simulink model "Alternative_VTOLAutopilotController"  (R2026a)
settings: configuration reference "VTOLConfiguration" (kept outside this file)
undefined symbols (not defined in the file): control, controlParams, ControlSampleTime, CriticalTiltAngle, DiscIntNeverNeededParam, dspblkCoreblockFVToolHelper, flightState, FSState, FWControlParams, FWTrimSpeed, gcbh, R_LOOKAHEAD, ReferenceFilterDen, ReferenceFilterNum, tilt_max, tilt_trim, tiltIni, TiltScheduleRate, uavParam, Vt, w_trim, WindDownRate, zGround
libraries: slpidlib x31, simulink x10, uavalgslib x7, simulink_extras x1, sl_discontinuities x1
(part 3 of 6)

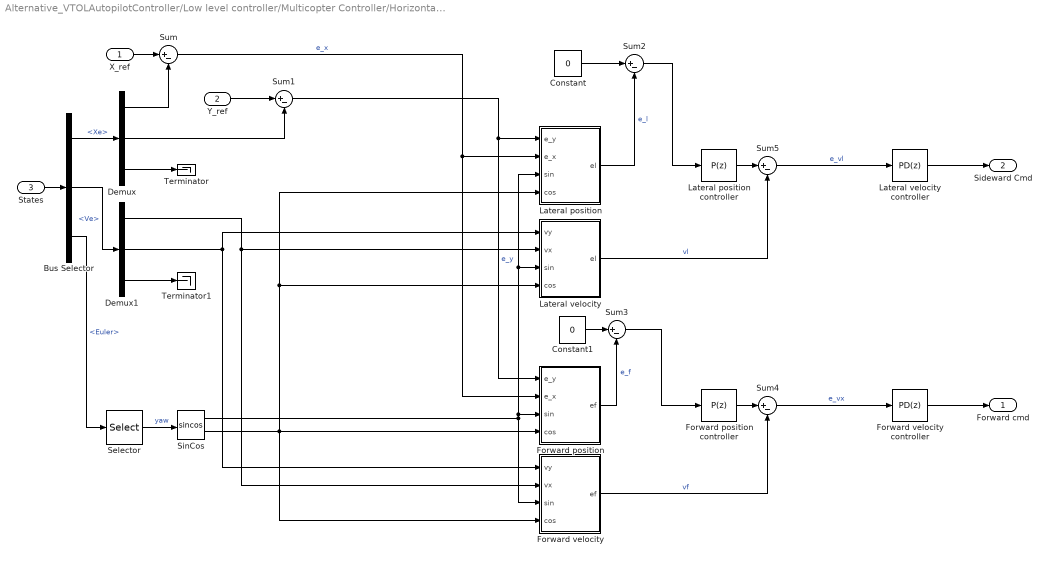
== system Alternative_VTOLAutopilotController/Low level controller/Multicopter Controller/Horizontal Position Control/XY Controller ==
  X_ref : Inport
  Y_ref : Inport  Port=2
  States : Inport  Port=3
  Bus Selector : BusSelector  OutputSignals=Xe,Ve,Euler
  Constant : Constant  Value=0
  Constant1 : Constant  Value=0
  Demux : Demux  Outputs=3
  Demux1 : Demux  Outputs=3
  Forward position : Subsystem
  Forward position controller : slpidlib/PID Controller  Controller=P  Form=Parallel  TimeDomain=Discrete-time  UseExternalTs=off  SampleTime=-1  IntegratorMethod=Forward Euler  FilterMethod=Forward Euler  ControllerParametersSource=internal  P=controlParams.P_X  I=controlParams.I_X  UseKiTs=off  D=0.741088334151374  UseExternalDerivativeSource=off  N=1.14081860742283  UseFilter=on  TunerSelectOption=Transfer Function Based (PID Tuner App)  InitialConditionSource=internal  InitialConditionForIntegrator=0  InitialConditionForFilter=0  DifferentiatorICPrevScaledInput=0  ExternalReset=none  TrackingMode=off  Kt=1  LimitOutput=off  SatLimitsSource=internal  UpperSaturationLimit=inf  LowerSaturationLimit=-inf  LinearizeAsGain=on  AntiWindupMode=none  Kb=1  LimitIntegrator=off  UpperIntegratorSaturationLimit=inf  LowerIntegratorSaturationLimit=-inf  POutMin=[]  POutMax=[]  IOutMin=[]  IOutMax=[]  DOutMin=[]  DOutMax=[]  NOutMin=[]  NOutMax=[]  SumOutMin=[]  SumOutMax=[]  SaturationOutMin=[]  SaturationOutMax=[]  PParamMin=[]  PParamMax=[]  IParamMin=[]  IParamMax=[]  DParamMin=[]  DParamMax=[]  NParamMin=[]  NParamMax=[]  KbParamMin=[]  KbParamMax=[]  KtParamMin=[]  KtParamMax=[]  KbOutMin=[]  KbOutMax=[]  KtOutMin=[]  KtOutMax=[]  IntegratorOutMin=[]  IntegratorOutMax=[]  FilterOutMin=[]  FilterOutMax=[]  SumI1OutMin=[]  SumI1OutMax=[]  SumI2OutMin=[]  SumI2OutMax=[]  SumI3OutMin=[]  SumI3OutMax=[]  SumI4OutMin=[]  SumI4OutMax=[]  SumDOutMin=[]  SumDOutMax=[]  DifferentiatorOutMin=[]  DifferentiatorOutMax=[]  FilterDiffOutCoefMin=[]  FilterDiffOutCoefMax=[]  ReciprocalOutMin=[]  ReciprocalOutMax=[]  SumDenOutMin=[]  SumDenOutMax=[]  SumNumOutMin=[]  SumNumOutMax=[]  DivideOutMin=[]  DivideOutMax=[]  UdiffTsProdOutMin=[]  UdiffTsProdOutMax=[]  NTsProdOutMin=[]  NTsProdOutMax=[]  UintegralTsProdOutMin=[]  UintegralTsProdOutMax=[]  UngainTsProdOutMin=[]  UngainTsProdOutMax=[]  ClampingZeroOutDataTypeStr=Inherit: Inherit via back propagation  ClampingZeroOutMin=[]  ClampingZeroOutMax=[]  FilterDenConstantOutDataTypeStr=Inherit: Inherit via back propagation  FilterDenConstantOutMin=[]  FilterDenConstantOutMax=[]  PCopyOutDataTypeStr=Inherit: Inherit via back propagation  PCopyOutMin=[]  PCopyOutMax=[]  NCopyOutDataTypeStr=Inherit: Inherit via back propagation  NCopyOutMin=[]  NCopyOutMax=[]  IntegratorContinuousStateAttributes=''  IntegratorStateMustResolveToSignalObject=off  IntegratorRTWStateStorageClass=Auto  FilterContinuousStateAttributes=''  FilterStateMustResolveToSignalObject=off  FilterRTWStateStorageClass=Auto  ParallelPVariant=InternalParameters  IdealPVariant=Disabled  IVariant=Disabled  DVariant=Disabled  IntegratorVariant=Disabled  SatVariant=Disabled  AWVariant=Disabled  PCopyVariant=Disabled  TRVariant=Disabled  FdbkBlocksVariant=Forward  IdealPFdbkVariant=Disabled  SatFdbkVariant=Disabled  DerivativeFilterVariant=Disabled  NVariant=Disabled  NCopyVariant=Disabled_SignalSpec  FilterICVariant=Disabled  IntegratorICVariant=Disabled  ExternalResetVariant=Disabled  TRSumVariant=Passthrough  SumFdbkVariant=Disabled  SumVariant=Passthrough_P  TsampFilterVariant=InternalTs  TsampNgainVariant=Passthrough  TsampIntegralVariant=Disabled_SignalSpec  ExternalSaturationOutDataTypeStr=Inherit: Same as second input  DerivativeSourceVariant=Disabled  PreIntVariant=InternalPreInt
  Forward velocity : Subsystem
  Forward velocity controller : slpidlib/PID Controller  Controller=PD  Form=Parallel  TimeDomain=Discrete-time  UseExternalTs=off  SampleTime=-1  IntegratorMethod=Forward Euler  FilterMethod=Forward Euler  ControllerParametersSource=internal  P=controlParams.P_VX  I=0  UseKiTs=off  D=controlParams.D_VX  UseExternalDerivativeSource=off  N=controlParams.N_VX  UseFilter=on  TunerSelectOption=Transfer Function Based (PID Tuner App)  InitialConditionSource=internal  InitialConditionForIntegrator=0  InitialConditionForFilter=0  DifferentiatorICPrevScaledInput=0  ExternalReset=none  TrackingMode=off  Kt=1  LimitOutput=off  SatLimitsSource=internal  UpperSaturationLimit=inf  LowerSaturationLimit=-inf  LinearizeAsGain=on  AntiWindupMode=none  Kb=1  LimitIntegrator=off  UpperIntegratorSaturationLimit=inf  LowerIntegratorSaturationLimit=-inf  POutMin=[]  POutMax=[]  IOutMin=[]  IOutMax=[]  DOutMin=[]  DOutMax=[]  NOutMin=[]  NOutMax=[]  SumOutMin=[]  SumOutMax=[]  SaturationOutMin=[]  SaturationOutMax=[]  PParamMin=[]  PParamMax=[]  IParamMin=[]  IParamMax=[]  DParamMin=[]  DParamMax=[]  NParamMin=[]  NParamMax=[]  KbParamMin=[]  KbParamMax=[]  KtParamMin=[]  KtParamMax=[]  KbOutMin=[]  KbOutMax=[]  KtOutMin=[]  KtOutMax=[]  IntegratorOutMin=[]  IntegratorOutMax=[]  FilterOutMin=[]  FilterOutMax=[]  SumI1OutMin=[]  SumI1OutMax=[]  SumI2OutMin=[]  SumI2OutMax=[]  SumI3OutMin=[]  SumI3OutMax=[]  SumI4OutMin=[]  SumI4OutMax=[]  SumDOutMin=[]  SumDOutMax=[]  DifferentiatorOutMin=[]  DifferentiatorOutMax=[]  FilterDiffOutCoefMin=[]  FilterDiffOutCoefMax=[]  ReciprocalOutMin=[]  ReciprocalOutMax=[]  SumDenOutMin=[]  SumDenOutMax=[]  SumNumOutMin=[]  SumNumOutMax=[]  DivideOutMin=[]  DivideOutMax=[]  UdiffTsProdOutMin=[]  UdiffTsProdOutMax=[]  NTsProdOutMin=[]  NTsProdOutMax=[]  UintegralTsProdOutMin=[]  UintegralTsProdOutMax=[]  UngainTsProdOutMin=[]  UngainTsProdOutMax=[]  ClampingZeroOutDataTypeStr=Inherit: Inherit via back propagation  ClampingZeroOutMin=[]  ClampingZeroOutMax=[]  FilterDenConstantOutDataTypeStr=Inherit: Inherit via back propagation  FilterDenConstantOutMin=[]  FilterDenConstantOutMax=[]  PCopyOutDataTypeStr=Inherit: Inherit via back propagation  PCopyOutMin=[]  PCopyOutMax=[]  NCopyOutDataTypeStr=Inherit: Inherit via back propagation  NCopyOutMin=[]  NCopyOutMax=[]  IntegratorContinuousStateAttributes=''  IntegratorStateMustResolveToSignalObject=off  IntegratorRTWStateStorageClass=Auto  FilterContinuousStateAttributes=''  FilterStateMustResolveToSignalObject=off  FilterRTWStateStorageClass=Auto  ParallelPVariant=InternalParameters  IdealPVariant=Disabled  IVariant=Disabled  DVariant=InternalParameters  IntegratorVariant=Disabled  SatVariant=Disabled  AWVariant=Disabled  PCopyVariant=Disabled  TRVariant=Disabled  FdbkBlocksVariant=Forward  IdealPFdbkVariant=Disabled  SatFdbkVariant=Disabled  DerivativeFilterVariant=ForwardEulerFilter  NVariant=InternalParameters  NCopyVariant=Disabled  FilterICVariant=InternalICsFilter  IntegratorICVariant=Disabled  ExternalResetVariant=Disabled  TRSumVariant=Passthrough  SumFdbkVariant=Disabled  SumVariant=Sum_PD  TsampFilterVariant=InternalTs  TsampNgainVariant=Passthrough  TsampIntegralVariant=Disabled_SignalSpec  ExternalSaturationOutDataTypeStr=Inherit: Same as second input  DerivativeSourceVariant=ErrorSignal  PreIntVariant=InternalPreInt
  Lateral position : Subsystem
  Lateral position controller : slpidlib/PID Controller  Controller=P  Form=Parallel  TimeDomain=Discrete-time  UseExternalTs=off  SampleTime=-1  IntegratorMethod=Forward Euler  FilterMethod=Forward Euler  ControllerParametersSource=internal  P=controlParams.P_Y  I=controlParams.I_Y  UseKiTs=off  D=0.20966837124708  UseExternalDerivativeSource=off  N=1.18305565097938  UseFilter=on  TunerSelectOption=Transfer Function Based (PID Tuner App)  InitialConditionSource=internal  InitialConditionForIntegrator=0  InitialConditionForFilter=0  DifferentiatorICPrevScaledInput=0  ExternalReset=none  TrackingMode=off  Kt=1  LimitOutput=off  SatLimitsSource=internal  UpperSaturationLimit=0.4  LowerSaturationLimit=-0.4  LinearizeAsGain=on  AntiWindupMode=clamping  Kb=1  LimitIntegrator=off  UpperIntegratorSaturationLimit=inf  LowerIntegratorSaturationLimit=-inf  POutMin=[]  POutMax=[]  IOutMin=[]  IOutMax=[]  DOutMin=[]  DOutMax=[]  NOutMin=[]  NOutMax=[]  SumOutMin=[]  SumOutMax=[]  SaturationOutMin=[]  SaturationOutMax=[]  PParamMin=[]  PParamMax=[]  IParamMin=[]  IParamMax=[]  DParamMin=[]  DParamMax=[]  NParamMin=[]  NParamMax=[]  KbParamMin=[]  KbParamMax=[]  KtParamMin=[]  KtParamMax=[]  KbOutMin=[]  KbOutMax=[]  KtOutMin=[]  KtOutMax=[]  IntegratorOutMin=[]  IntegratorOutMax=[]  FilterOutMin=[]  FilterOutMax=[]  SumI1OutMin=[]  SumI1OutMax=[]  SumI2OutMin=[]  SumI2OutMax=[]  SumI3OutMin=[]  SumI3OutMax=[]  SumI4OutMin=[]  SumI4OutMax=[]  SumDOutMin=[]  SumDOutMax=[]  DifferentiatorOutMin=[]  DifferentiatorOutMax=[]  FilterDiffOutCoefMin=[]  FilterDiffOutCoefMax=[]  ReciprocalOutMin=[]  ReciprocalOutMax=[]  SumDenOutMin=[]  SumDenOutMax=[]  SumNumOutMin=[]  SumNumOutMax=[]  DivideOutMin=[]  DivideOutMax=[]  UdiffTsProdOutMin=[]  UdiffTsProdOutMax=[]  NTsProdOutMin=[]  NTsProdOutMax=[]  UintegralTsProdOutMin=[]  UintegralTsProdOutMax=[]  UngainTsProdOutMin=[]  UngainTsProdOutMax=[]  ClampingZeroOutDataTypeStr=Inherit: Inherit via back propagation  ClampingZeroOutMin=[]  ClampingZeroOutMax=[]  FilterDenConstantOutDataTypeStr=Inherit: Inherit via back propagation  FilterDenConstantOutMin=[]  FilterDenConstantOutMax=[]  PCopyOutDataTypeStr=Inherit: Inherit via back propagation  PCopyOutMin=[]  PCopyOutMax=[]  NCopyOutDataTypeStr=Inherit: Inherit via back propagation  NCopyOutMin=[]  NCopyOutMax=[]  IntegratorContinuousStateAttributes=''  IntegratorStateMustResolveToSignalObject=off  IntegratorRTWStateStorageClass=Auto  FilterContinuousStateAttributes=''  FilterStateMustResolveToSignalObject=off  FilterRTWStateStorageClass=Auto  ParallelPVariant=InternalParameters  IdealPVariant=Disabled  IVariant=Disabled  DVariant=Disabled  IntegratorVariant=Disabled  SatVariant=Disabled  AWVariant=Disabled  PCopyVariant=Disabled  TRVariant=Disabled  FdbkBlocksVariant=Forward  IdealPFdbkVariant=Disabled  SatFdbkVariant=Disabled  DerivativeFilterVariant=Disabled  NVariant=Disabled  NCopyVariant=Disabled_SignalSpec  FilterICVariant=Disabled  IntegratorICVariant=Disabled  ExternalResetVariant=Disabled  TRSumVariant=Passthrough  SumFdbkVariant=Disabled  SumVariant=Passthrough_P  TsampFilterVariant=InternalTs  TsampNgainVariant=Passthrough  TsampIntegralVariant=Disabled_SignalSpec  ExternalSaturationOutDataTypeStr=Inherit: Same as second input  DerivativeSourceVariant=Disabled  PreIntVariant=InternalPreInt
  Lateral velocity : Subsystem
  "Lateral velocity controller " : slpidlib/PID Controller  Controller=PD  Form=Parallel  TimeDomain=Discrete-time  UseExternalTs=off  SampleTime=-1  IntegratorMethod=Forward Euler  FilterMethod=Forward Euler  ControllerParametersSource=internal  P=controlParams.P_VY  I=0  UseKiTs=off  D=controlParams.D_VY  UseExternalDerivativeSource=off  N=controlParams.N_VY  UseFilter=on  TunerSelectOption=Transfer Function Based (PID Tuner App)  InitialConditionSource=internal  InitialConditionForIntegrator=0  InitialConditionForFilter=0  DifferentiatorICPrevScaledInput=0  ExternalReset=none  TrackingMode=off  Kt=1  LimitOutput=off  SatLimitsSource=internal  UpperSaturationLimit=inf  LowerSaturationLimit=-inf  LinearizeAsGain=on  AntiWindupMode=none  Kb=1  LimitIntegrator=off  UpperIntegratorSaturationLimit=inf  LowerIntegratorSaturationLimit=-inf  POutMin=[]  POutMax=[]  IOutMin=[]  IOutMax=[]  DOutMin=[]  DOutMax=[]  NOutMin=[]  NOutMax=[]  SumOutMin=[]  SumOutMax=[]  SaturationOutMin=[]  SaturationOutMax=[]  PParamMin=[]  PParamMax=[]  IParamMin=[]  IParamMax=[]  DParamMin=[]  DParamMax=[]  NParamMin=[]  NParamMax=[]  KbParamMin=[]  KbParamMax=[]  KtParamMin=[]  KtParamMax=[]  KbOutMin=[]  KbOutMax=[]  KtOutMin=[]  KtOutMax=[]  IntegratorOutMin=[]  IntegratorOutMax=[]  FilterOutMin=[]  FilterOutMax=[]  SumI1OutMin=[]  SumI1OutMax=[]  SumI2OutMin=[]  SumI2OutMax=[]  SumI3OutMin=[]  SumI3OutMax=[]  SumI4OutMin=[]  SumI4OutMax=[]  SumDOutMin=[]  SumDOutMax=[]  DifferentiatorOutMin=[]  DifferentiatorOutMax=[]  FilterDiffOutCoefMin=[]  FilterDiffOutCoefMax=[]  ReciprocalOutMin=[]  ReciprocalOutMax=[]  SumDenOutMin=[]  SumDenOutMax=[]  SumNumOutMin=[]  SumNumOutMax=[]  DivideOutMin=[]  DivideOutMax=[]  UdiffTsProdOutMin=[]  UdiffTsProdOutMax=[]  NTsProdOutMin=[]  NTsProdOutMax=[]  UintegralTsProdOutMin=[]  UintegralTsProdOutMax=[]  UngainTsProdOutMin=[]  UngainTsProdOutMax=[]  ClampingZeroOutDataTypeStr=Inherit: Inherit via back propagation  ClampingZeroOutMin=[]  ClampingZeroOutMax=[]  FilterDenConstantOutDataTypeStr=Inherit: Inherit via back propagation  FilterDenConstantOutMin=[]  FilterDenConstantOutMax=[]  PCopyOutDataTypeStr=Inherit: Inherit via back propagation  PCopyOutMin=[]  PCopyOutMax=[]  NCopyOutDataTypeStr=Inherit: Inherit via back propagation  NCopyOutMin=[]  NCopyOutMax=[]  IntegratorContinuousStateAttributes=''  IntegratorStateMustResolveToSignalObject=off  IntegratorRTWStateStorageClass=Auto  FilterContinuousStateAttributes=''  FilterStateMustResolveToSignalObject=off  FilterRTWStateStorageClass=Auto  ParallelPVariant=InternalParameters  IdealPVariant=Disabled  IVariant=Disabled  DVariant=InternalParameters  IntegratorVariant=Disabled  SatVariant=Disabled  AWVariant=Disabled  PCopyVariant=Disabled  TRVariant=Disabled  FdbkBlocksVariant=Forward  IdealPFdbkVariant=Disabled  SatFdbkVariant=Disabled  DerivativeFilterVariant=ForwardEulerFilter  NVariant=InternalParameters  NCopyVariant=Disabled  FilterICVariant=InternalICsFilter  IntegratorICVariant=Disabled  ExternalResetVariant=Disabled  TRSumVariant=Passthrough  SumFdbkVariant=Disabled  SumVariant=Sum_PD  TsampFilterVariant=InternalTs  TsampNgainVariant=Passthrough  TsampIntegralVariant=Disabled_SignalSpec  ExternalSaturationOutDataTypeStr=Inherit: Same as second input  DerivativeSourceVariant=ErrorSignal  PreIntVariant=InternalPreInt
  Selector : Selector  InputPortWidth=3  IndexOptions=Index vector (dialog)  Indices=[3]  OutputSizes=1
  SinCos : Trigonometry  Operator=sincos
  Sum{,1..5} (6 alike) : Sum  Inputs=|+-
  Terminator : Terminator
  Terminator1 : Terminator
  Forward cmd : Outport
  Sideward Cmd : Outport  Port=2
  wires:
  Demux/1 -> Sum/2
  States/1 -> Bus Selector/1
  Bus Selector/1 -> Demux/1  "<Xe>"
  X_ref/1 -> Sum/1
  Bus Selector/2 -> Demux1/1  "<Ve>"
  Y_ref/1 -> Sum1/1
  Demux/2 -> Sum1/2
  Demux/3 -> Terminator/1
  Sum4/1 -> Forward velocity controller/1  "e_vx"
  SinCos/2 -> Forward velocity/4(cos), Lateral position/4(cos), Lateral velocity/4(cos), Forward position/4(cos)
  Selector/1 -> SinCos/1  "yaw"
  Lateral position/1(el) -> Sum2/2  "e_l"
  Sum1/1 -> Forward position/1(e_y), Lateral position/1(e_y)  "e_y"
  Sum/1 -> Forward position/2(e_x), Lateral position/2(e_x)  "e_x"
  Demux1/1 -> Forward velocity/2(vx), Lateral velocity/2(vx)
  Demux1/2 -> Forward velocity/1(vy), Lateral velocity/1(vy)
  Demux1/3 -> Terminator1/1
  SinCos/1 -> Lateral velocity/3(sin), Lateral position/3(sin), Forward position/3(sin), Forward velocity/3(sin)
  Lateral velocity/1(el) -> Sum5/2  "vl"
  Forward position/1(ef) -> Sum3/2  "e_f"
  Forward velocity/1(ef) -> Sum4/2  "vf"
  Lateral position controller/1 -> Sum5/1
  Forward position controller/1 -> Sum4/1
  Sum5/1 -> "Lateral velocity controller "/1  "e_vl"
  Bus Selector/3 -> Selector/1  "<Euler>"
  "Lateral velocity controller "/1 -> Sideward Cmd/1
  Forward velocity controller/1 -> Forward cmd/1
  Constant/1 -> Sum2/1
  Sum2/1 -> Lateral position controller/1
  Constant1/1 -> Sum3/1
  Sum3/1 -> Forward position controller/1

== system Alternative_VTOLAutopilotController/Low level controller/Multicopter Controller/Subsystem/Triggered Subsystem ==
  YawHold : Inport
  Trigger : TriggerPort  VariantControl=(inherit)
  Reference : Outport
  wires:
  YawHold/1 -> Reference/1

== system Alternative_VTOLAutopilotController/Low level controller/Scheduler/FixedWingScheduler/Switch Case Action Subsystem ==
  note: No control allocated from fixed wing during hover.
  Action Port : ActionPort  ActionPortLabel=case [ Hover ]:
  Bus Creator : BusCreator  Inputs=4
  Constant{,1..3} (4 alike) : Constant  Value=0
  FixedWingControls : Outport  OutDataTypeStr=Bus: FixedWingCtrlBus
  wires:
  Bus Creator/1 -> FixedWingControls/1
  Constant/1 -> Bus Creator/1  "dA"
  Constant1/1 -> Bus Creator/2  "dE"
  Constant2/1 -> Bus Creator/3  "dR"
  Constant3/1 -> Bus Creator/4  "dT"

== system Alternative_VTOLAutopilotController/Low level controller/Scheduler/FixedWingScheduler/Switch Case Action Subsystem1 ==
  FixedWingActuators : Inport  OutDataTypeStr=Bus: FixedWingCtrlBus
  TransitionDone : Inport  Port=2
  Action Port : ActionPort  ActionPortLabel=case [ Transition ]:
  Bus Creator : BusCreator  Inputs=4  OutDataTypeStr=Bus: FixedWingCtrlBus
  Constant : Constant  Value=0
  Constant1 : Constant  Value=-0.2
  Constant2 : Constant  Value=0
  Constant3 : Constant  Value=0
  Switch : Switch  Criteria=u2 > Threshold  SaturateOnIntegerOverflow=off  InputSameDT=off
  FixedWingControls : Outport  OutDataTypeStr=Bus: FixedWingCtrlBus
  wires:
  Bus Creator/1 -> Switch/3
  Constant/1 -> Bus Creator/1  "dA"
  Constant1/1 -> Bus Creator/2  "dE"
  Constant2/1 -> Bus Creator/3  "dR"
  Constant3/1 -> Bus Creator/4  "dT"
  FixedWingActuators/1 -> Switch/1
  Switch/1 -> FixedWingControls/1
  TransitionDone/1 -> Switch/2

== system Alternative_VTOLAutopilotController/Low level controller/Scheduler/FixedWingScheduler/Switch Case Action Subsystem2 ==
  FixedWingActuators : Inport  OutDataTypeStr=Bus: FixedWingCtrlBus
  Action Port : ActionPort  ActionPortLabel=case [ FixedWing ]:
  FixedWingControls : Outport  OutDataTypeStr=Bus: FixedWingCtrlBus
  wires:
  FixedWingActuators/1 -> FixedWingControls/1

== system Alternative_VTOLAutopilotController/Low level controller/Scheduler/FixedWingScheduler/Switch Case Action Subsystem3 ==
  note: No control allocated from fixed wing during hover.
  Action Port : ActionPort  ActionPortLabel=case [ BackTransition ]:
  Bus Creator : BusCreator  Inputs=4
  Constant{,1..3} (4 alike) : Constant  Value=0
  FixedWingControls : Outport  OutDataTypeStr=Bus: FixedWingCtrlBus
  wires:
  Bus Creator/1 -> FixedWingControls/1
  Constant/1 -> Bus Creator/1  "dA"
  Constant1/1 -> Bus Creator/2  "dE"
  Constant3/1 -> Bus Creator/4  "dT"
  Constant2/1 -> Bus Creator/3  "dR"

== system Alternative_VTOLAutopilotController/Low level controller/Scheduler/Subsystem/Actuator To Voltage ==
  Motor Commands : Inport
  Bus Creator : BusCreator  Inputs=9  OutDataTypeStr=Bus: RotorCtrlBus
  Bus Selector : BusSelector  OutputSignals=w1,w2,w3,w4,Tilt1,Tilt2,Tilt3,Tilt4,w5
  Gain{,1..2,4,8} (5 alike) : Gain  Gain=1/(uavParam.motor.RPMMAX/60)
  Gain{3,5..7} (4 alike) : Gain  Gain=1/(pi/2)
  To PWM : Outport
  wires:
  Motor Commands/1 -> Bus Selector/1
  Bus Selector/1 -> Gain/1  "<w1>"
  Bus Selector/3 -> Gain1/1  "<w3>"
  Bus Selector/2 -> Gain4/1  "<w2>"
  Bus Selector/4 -> Gain2/1  "<w4>"
  Bus Selector/5 -> Gain3/1  "<Tilt1>"
  Bus Selector/6 -> Gain5/1  "<Tilt2>"
  Gain/1 -> Bus Creator/1  "w1"
  Gain4/1 -> Bus Creator/2  "w2"
  Gain1/1 -> Bus Creator/3  "w3"
  Gain2/1 -> Bus Creator/4  "w4"
  Gain3/1 -> Bus Creator/5  "Tilt1"
  Gain5/1 -> Bus Creator/6  "Tilt2"
  Bus Creator/1 -> To PWM/1
  Bus Selector/8 -> Gain7/1  "<Tilt4>"
  Gain7/1 -> Bus Creator/8  "Tilt4"
  Bus Selector/7 -> Gain6/1  "<Tilt3>"
  Gain6/1 -> Bus Creator/7  "Tilt3"
  Gain8/1 -> Bus Creator/9  "w5"
  Bus Selector/9 -> Gain8/1  "<w5>"

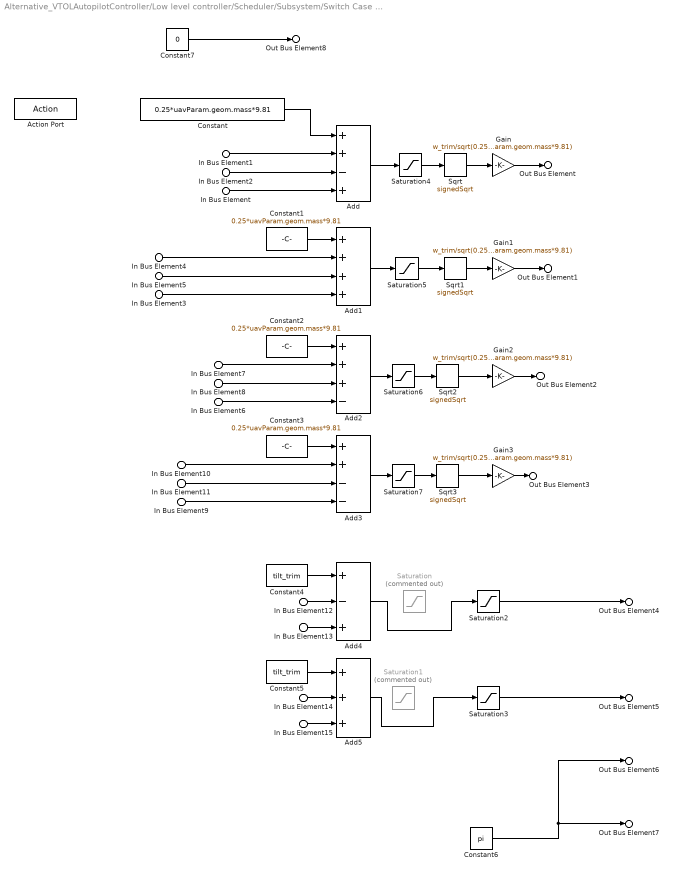
== system Alternative_VTOLAutopilotController/Low level controller/Scheduler/Subsystem/Switch Case Action Subsystem ==
  In Bus Element{,3,6,9} (4 alike) : Inport  PortName=MixerCommands  Element=w_theta
  In Bus Element{1,4,7,10} (4 alike) : Inport  PortName=MixerCommands  Element=w_z
  In Bus Element{2,5,8,11} (4 alike) : Inport  PortName=MixerCommands  Element=w_phi
  In Bus Element12 : Inport  PortName=MixerCommands  Element=l_psi
  In Bus Element14 : Inport  PortName=MixerCommands  Element=l_psi
  In Bus Element13 : Inport  PortName=MixerCommands  Element=l_x
  In Bus Element15 : Inport  PortName=MixerCommands  Element=l_x
  Action Port : ActionPort  ActionPortLabel=case [ Hover ]:
  Add : Sum  Inputs=++-+
  Add1 : Sum  Inputs=++++
  Add2 : Sum  Inputs=+++-
  Add3 : Sum  Inputs=++--
  Add4 : Sum  Inputs=+-+
  Add5 : Sum  Inputs=+++
  Constant{,1..3} (4 alike) : Constant  Value=0.25*uavParam.geom.mass*9.81
  Constant4 : Constant  Value=tilt_trim
  Constant5 : Constant  Value=tilt_trim
  Constant6 : Constant  Value=pi
  Constant7 : Constant  Value=0
  Gain{,1..3} (4 alike) : Gain  Gain=w_trim/sqrt(0.25*uavParam.geom.mass*9.81)
  Saturation : Saturate  Commented=on  UpperLimit=tilt_max  LowerLimit=-tilt_max
  Saturation1 : Saturate  Commented=on  UpperLimit=tilt_max  LowerLimit=-tilt_max
  Saturation2 : Saturate  UpperLimit=tilt_max  LowerLimit=-tilt_max
  Saturation3 : Saturate  UpperLimit=tilt_max  LowerLimit=-tilt_max
  Saturation{4..7} (4 alike) : Saturate  UpperLimit=inf  LowerLimit=0
  Sqrt{,1..3} (4 alike) : Sqrt  Operator=signedSqrt
  Out Bus Element : Outport  PortName=Actuator  Element=w1
  Out Bus Element1 : Outport  PortName=Actuator  Element=w2
  Out Bus Element2 : Outport  PortName=Actuator  Element=w3
  Out Bus Element3 : Outport  PortName=Actuator  Element=w4
  Out Bus Element4 : Outport  PortName=Actuator  Element=Tilt1
  Out Bus Element5 : Outport  PortName=Actuator  Element=Tilt2
  Out Bus Element6 : Outport  PortName=Actuator  Element=Tilt3
  Out Bus Element7 : Outport  PortName=Actuator  Element=Tilt4
  Out Bus Element8 : Outport  PortName=Actuator  Element=w5
  wires:
  Constant5/1 -> Add5/1
  Constant2/1 -> Add2/1
  Constant1/1 -> Add1/1
  Constant4/1 -> Add4/1
  Constant/1 -> Add/1
  Constant3/1 -> Add3/1
  Add/1 -> Saturation4/1
  Add1/1 -> Saturation5/1
  Add2/1 -> Saturation6/1
  Add3/1 -> Saturation7/1
  In Bus Element12/1 -> Add4/2
  In Bus Element13/1 -> Add4/3
  In Bus Element14/1 -> Add5/2
  In Bus Element15/1 -> Add5/3
  Saturation2/1 -> Out Bus Element4/1
  Add4/1 -> Saturation2/1
  Add5/1 -> Saturation3/1
  Saturation3/1 -> Out Bus Element5/1
  Sqrt1/1 -> Gain1/1
  Sqrt2/1 -> Gain2/1
  Sqrt3/1 -> Gain3/1
  Saturation4/1 -> Sqrt/1
  Saturation5/1 -> Sqrt1/1
  Saturation6/1 -> Sqrt2/1
  Saturation7/1 -> Sqrt3/1
  Sqrt/1 -> Gain/1
  Gain/1 -> Out Bus Element/1
  Gain1/1 -> Out Bus Element1/1
  Gain2/1 -> Out Bus Element2/1
  Gain3/1 -> Out Bus Element3/1
  In Bus Element2/1 -> Add/3
  In Bus Element1/1 -> Add/2
  In Bus Element/1 -> Add/4
  In Bus Element4/1 -> Add1/2
  In Bus Element5/1 -> Add1/3
  In Bus Element3/1 -> Add1/4
  In Bus Element7/1 -> Add2/2
  In Bus Element8/1 -> Add2/3
  In Bus Element10/1 -> Add3/2
  In Bus Element11/1 -> Add3/3
  In Bus Element9/1 -> Add3/4
  In Bus Element6/1 -> Add2/4
  Constant6/1 -> Out Bus Element7/1, Out Bus Element6/1
  Constant7/1 -> Out Bus Element8/1

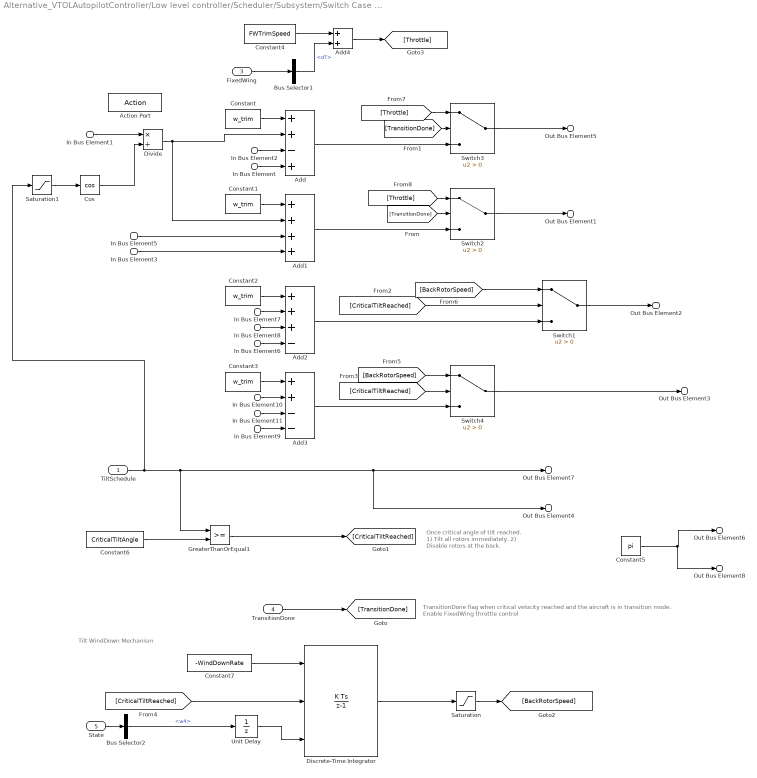
== system Alternative_VTOLAutopilotController/Low level controller/Scheduler/Subsystem/Switch Case Action Subsystem1 ==
  note: Tilt WindDown Mechanism
  note: Once critical angle of tilt reached.
      | 1) Tilt all rotors immediately.
      | 2) Disable rotors at the back.
  note: TransitionDone flag when critical velocity reached and the aircraft is in transition mode.
      | Enable FixedWing throttle control
  TiltSchedule : Inport
  In Bus Element{,3,6,9} (4 alike) : Inport  Port=2  PortName=MixerCommands  Element=w_theta
  In Bus Element1 : Inport  Port=2  PortName=MixerCommands  Element=w_z
  In Bus Element7 : Inport  Port=2  PortName=MixerCommands  Element=w_z
  In Bus Element10 : Inport  Port=2  PortName=MixerCommands  Element=w_z
  In Bus Element{2,5,8,11} (4 alike) : Inport  Port=2  PortName=MixerCommands  Element=w_phi
  FixedWing : Inport  Port=3
  TransitionDone : Inport  Port=4
  State : Inport  Port=5
  Action Port : ActionPort  ActionPortLabel=case [ Transition ]:
  Add : Sum  Inputs=++-+
  Add1 : Sum  Inputs=++++
  Add2 : Sum  Inputs=+++-
  Add3 : Sum  Inputs=++--
  Add4 : Sum
  Bus Selector1 : BusSelector  OutputSignals=dT
  Bus Selector2 : BusSelector  OutputSignals=RotorParameters.w4
  Constant{,1..3} (4 alike) : Constant  Value=w_trim
  Constant4 : Constant  Value=FWTrimSpeed
  Constant5 : Constant  Value=pi
  Constant6 : Constant  Value=CriticalTiltAngle
  Constant7 : Constant  Value=-WindDownRate
  Cos : Trigonometry  Operator=cos
  Discrete-Time Integrator : DiscreteIntegrator  ExternalReset=either  InitialConditionSource=external  SampleTime=0.005  ICPrevOutput=DiscIntNeverNeededParam  ICPrevScaledInput=DiscIntNeverNeededParam
  Divide : Product  Inputs=*/
  GreaterThanOrEqual1 : RelationalOperator  OutDataTypeStr=boolean  RndMeth=Simplest  InputSameDT=off
  Saturation : Saturate  UpperLimit=Inf  LowerLimit=0
  Saturation1 : Saturate  UpperLimit=CriticalTiltAngle  LowerLimit=-CriticalTiltAngle
  Switch{1..4} (4 alike) : Switch  Criteria=u2 > Threshold  SaturateOnIntegerOverflow=off  InputSameDT=off
  Unit Delay : UnitDelay  SampleTime=-1
  Out Bus Element5 : Outport  PortName=Actuator  Element=w1
  Out Bus Element1 : Outport  PortName=Actuator  Element=w2
  Out Bus Element2 : Outport  PortName=Actuator  Element=w3
  Out Bus Element3 : Outport  PortName=Actuator  Element=w4
  Out Bus Element7 : Outport  PortName=Actuator  Element=Tilt1
  Out Bus Element4 : Outport  PortName=Actuator  Element=Tilt2
  Out Bus Element6 : Outport  PortName=Actuator  Element=Tilt3
  Out Bus Element8 : Outport  PortName=Actuator  Element=Tilt4
  wires:
  TiltSchedule/1 -> GreaterThanOrEqual1/1, Out Bus Element4/1, Out Bus Element7/1, Saturation1/1
  In Bus Element9/1 -> Add3/4
  In Bus Element6/1 -> Add2/4
  In Bus Element8/1 -> Add2/3
  Constant3/1 -> Add3/1
  In Bus Element/1 -> Add/4
  In Bus Element10/1 -> Add3/2
  Constant1/1 -> Add1/1
  In Bus Element11/1 -> Add3/3
  In Bus Element3/1 -> Add1/4
  In Bus Element2/1 -> Add/3
  In Bus Element7/1 -> Add2/2
  Constant2/1 -> Add2/1
  In Bus Element5/1 -> Add1/3
  Constant/1 -> Add/1
  [TransitionDone] -> Switch2/2
  FixedWing/1 -> Bus Selector1/1
  Bus Selector1/1 -> Add4/2  "<dT>"
  [TransitionDone] -> Switch3/2
  Constant6/1 -> GreaterThanOrEqual1/2
  GreaterThanOrEqual1/1 -> [CriticalTiltReached]
  [CriticalTiltReached] -> Switch1/2
  Add2/1 -> Switch1/3
  [BackRotorSpeed] -> Switch1/1
  [CriticalTiltReached] -> Switch4/2
  Add3/1 -> Switch4/3
  [BackRotorSpeed] -> Switch4/1
  TransitionDone/1 -> [TransitionDone]
  Bus Selector2/1 -> Unit Delay/1  "<w4>"
  Constant7/1 -> Discrete-Time Integrator/1
  [CriticalTiltReached] -> Discrete-Time Integrator/2
  Discrete-Time Integrator/1 -> Saturation/1
  Saturation/1 -> [BackRotorSpeed]
  State/1 -> Bus Selector2/1
  Unit Delay/1 -> Discrete-Time Integrator/3
  Constant4/1 -> Add4/1
  Add4/1 -> [Throttle]
  [Throttle] -> Switch3/1
  [Throttle] -> Switch2/1
  Add/1 -> Switch3/3
  Cos/1 -> Divide/2
  Add1/1 -> Switch2/3
  Saturation1/1 -> Cos/1
  In Bus Element1/1 -> Divide/1
  Divide/1 -> Add1/2, Add/2
  Switch3/1 -> Out Bus Element5/1
  Switch2/1 -> Out Bus Element1/1
  Switch1/1 -> Out Bus Element2/1
  Switch4/1 -> Out Bus Element3/1
  Constant5/1 -> Out Bus Element8/1, Out Bus Element6/1

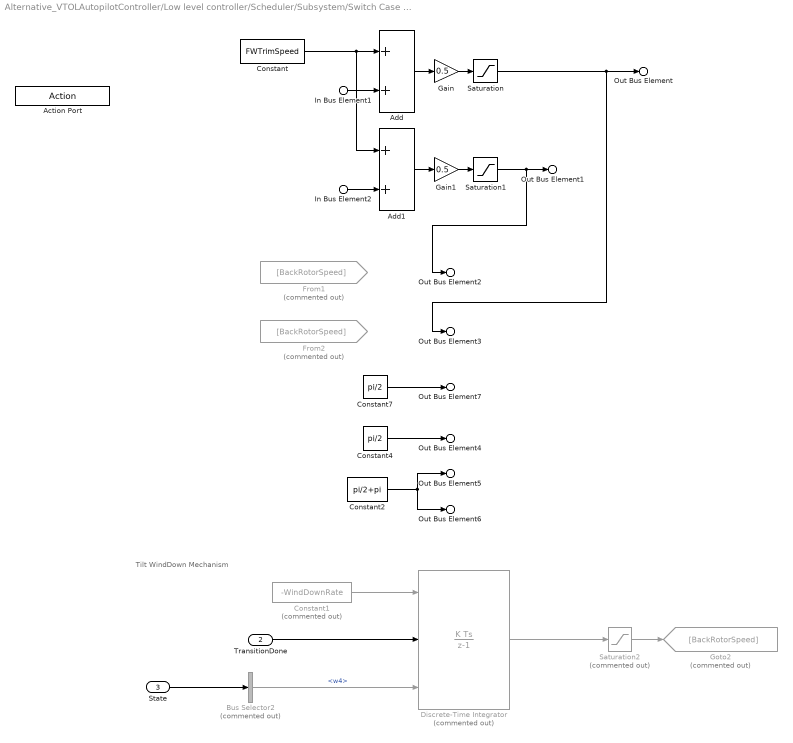
== system Alternative_VTOLAutopilotController/Low level controller/Scheduler/Subsystem/Switch Case Action Subsystem2 ==
  note: Tilt WindDown Mechanism
  In Bus Element2 : Inport  PortName=FixedWingCtrlBus  Element=dT
  In Bus Element1 : Inport  PortName=FixedWingCtrlBus  Element=dT
  TransitionDone : Inport  Port=2
  State : Inport  Port=3
  Action Port : ActionPort  ActionPortLabel=case [ FixedWing ]:
  Add : Sum
  Add1 : Sum
  Bus Selector2 : BusSelector  Commented=on  OutputSignals=RotorParameters.w4
  Constant : Constant  Value=FWTrimSpeed
  Constant1 : Constant  Commented=on  Value=-WindDownRate
  Constant2 : Constant  Value=pi/2+pi
  Constant4 : Constant  Value=pi/2
  Constant7 : Constant  Value=pi/2
  Discrete-Time Integrator : DiscreteIntegrator  Commented=on  ExternalReset=rising  InitialConditionSource=external  SampleTime=0.005  ICPrevOutput=DiscIntNeverNeededParam  ICPrevScaledInput=DiscIntNeverNeededParam
  From1 : From  Commented=on  GotoTag=BackRotorSpeed
  From2 : From  Commented=on  GotoTag=BackRotorSpeed
  Gain : Gain  Gain=0.5
  Gain1 : Gain  Gain=0.5
  Goto2 : Goto  Commented=on  GotoTag=BackRotorSpeed
  Saturation : Saturate  UpperLimit=Inf  LowerLimit=0
  Saturation1 : Saturate  UpperLimit=Inf  LowerLimit=0
  Saturation2 : Saturate  Commented=on  UpperLimit=Inf  LowerLimit=0
  Out Bus Element : Outport  PortName=Actuator  Element=w1
  Out Bus Element1 : Outport  PortName=Actuator  Element=w2
  Out Bus Element2 : Outport  PortName=Actuator  Element=w3
  Out Bus Element3 : Outport  PortName=Actuator  Element=w4
  Out Bus Element7 : Outport  PortName=Actuator  Element=Tilt1
  Out Bus Element4 : Outport  PortName=Actuator  Element=Tilt2
  Out Bus Element5 : Outport  PortName=Actuator  Element=Tilt3
  Out Bus Element6 : Outport  PortName=Actuator  Element=Tilt4
  wires:
  Add1/1 -> Gain1/1
  Constant4/1 -> Out Bus Element4/1
  Constant/1 -> Add1/1, Add/1
  Constant7/1 -> Out Bus Element7/1
  In Bus Element2/1 -> Add1/2
  Add/1 -> Gain/1
  In Bus Element1/1 -> Add/2
  Bus Selector2/1 -> Discrete-Time Integrator/3  "<w4>"
  Saturation2/1 -> Goto2/1
  State/1 -> Bus Selector2/1
  Constant1/1 -> Discrete-Time Integrator/1
  Discrete-Time Integrator/1 -> Saturation2/1
  TransitionDone/1 -> Discrete-Time Integrator/2
  Saturation/1 -> Out Bus Element3/1, Out Bus Element/1
  Saturation1/1 -> Out Bus Element2/1, Out Bus Element1/1
  Constant2/1 -> Out Bus Element5/1, Out Bus Element6/1
  Gain/1 -> Saturation/1
  Gain1/1 -> Saturation1/1

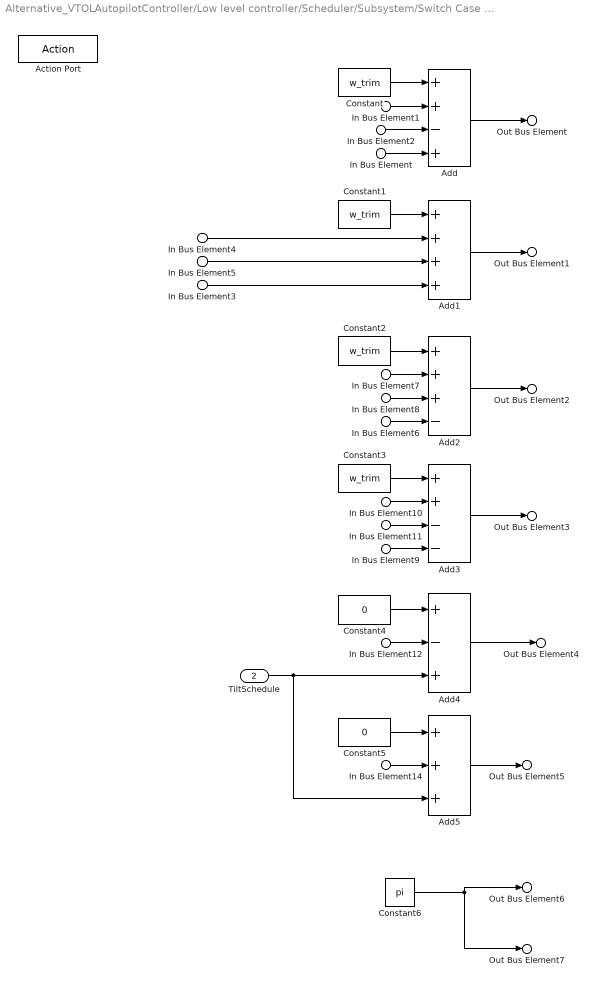
== system Alternative_VTOLAutopilotController/Low level controller/Scheduler/Subsystem/Switch Case Action Subsystem3 ==
  In Bus Element{,3,6,9} (4 alike) : Inport  PortName=MixerCommands  Element=w_theta
  In Bus Element{1,4,7,10} (4 alike) : Inport  PortName=MixerCommands  Element=w_z
  In Bus Element{2,5,8,11} (4 alike) : Inport  PortName=MixerCommands  Element=w_phi
  In Bus Element12 : Inport  PortName=MixerCommands  Element=l_psi
  In Bus Element14 : Inport  PortName=MixerCommands  Element=l_psi
  TiltSchedule : Inport  Port=2
  Action Port : ActionPort  ActionPortLabel=case [ BackTransition ]:
  Add : Sum  Inputs=++-+
  Add1 : Sum  Inputs=++++
  Add2 : Sum  Inputs=+++-
  Add3 : Sum  Inputs=++--
  Add4 : Sum  Inputs=+-+
  Add5 : Sum  Inputs=+++
  Constant{,1..3} (4 alike) : Constant  Value=w_trim
  Constant4 : Constant  Value=0
  Constant5 : Constant  Value=0
  Constant6 : Constant  Value=pi
  Out Bus Element : Outport  PortName=Actuator  Element=w1
  Out Bus Element1 : Outport  PortName=Actuator  Element=w2
  Out Bus Element2 : Outport  PortName=Actuator  Element=w3
  Out Bus Element3 : Outport  PortName=Actuator  Element=w4
  Out Bus Element4 : Outport  PortName=Actuator  Element=Tilt1
  Out Bus Element5 : Outport  PortName=Actuator  Element=Tilt2
  Out Bus Element6 : Outport  PortName=Actuator  Element=Tilt3
  Out Bus Element7 : Outport  PortName=Actuator  Element=Tilt4
  wires:
  In Bus Element4/1 -> Add1/2
  In Bus Element2/1 -> Add/3
  In Bus Element5/1 -> Add1/3
  In Bus Element3/1 -> Add1/4
  In Bus Element/1 -> Add/4
  In Bus Element11/1 -> Add3/3
  In Bus Element8/1 -> Add2/3
  Constant2/1 -> Add2/1
  In Bus Element9/1 -> Add3/4
  In Bus Element6/1 -> Add2/4
  Constant1/1 -> Add1/1
  In Bus Element10/1 -> Add3/2
  In Bus Element1/1 -> Add/2
  Add1/1 -> Out Bus Element1/1
  Constant/1 -> Add/1
  Constant3/1 -> Add3/1
  Add/1 -> Out Bus Element/1
  Add2/1 -> Out Bus Element2/1
  Add3/1 -> Out Bus Element3/1
  In Bus Element7/1 -> Add2/2
  Constant4/1 -> Add4/1
  In Bus Element12/1 -> Add4/2
  TiltSchedule/1 -> Add5/3, Add4/3
  Constant5/1 -> Add5/1
  In Bus Element14/1 -> Add5/2
  Add4/1 -> Out Bus Element4/1
  Add5/1 -> Out Bus Element5/1
  Constant6/1 -> Out Bus Element6/1, Out Bus Element7/1

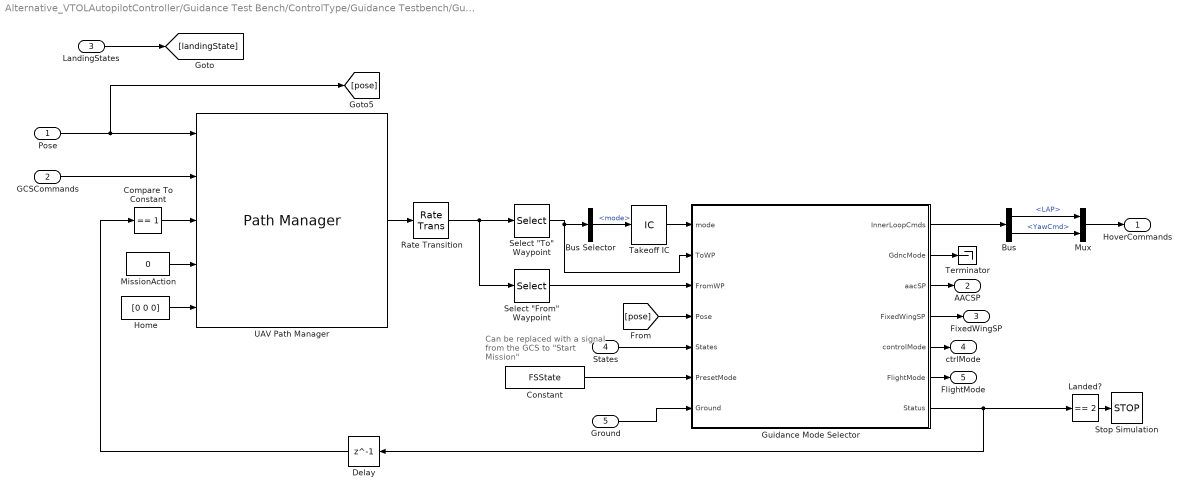
== system Alternative_VTOLAutopilotController/Guidance Test Bench/ControlType/Guidance Testbench/Guidance Logic/Guidance Stateflow ==
  note: Can be replaced with a signal from the GCS to "Start Mission"
  Pose : Inport
  GCSCommands : Inport  Port=2
  LandingStates : Inport  Port=3
  States : Inport  Port=4
  Ground : Inport  Port=5
  "Bus " : BusSelector  OutputSignals=LAP,YawCmd
  Bus Selector : BusSelector  OutputSignals=mode
  Compare To Constant : simulink/Logic and Bit Operations/Compare To Constant  relop===  const=1  OutDataTypeStr=boolean
  Constant : Constant  Value=FSState
  Delay : Delay  DelayLength=1  InitialCondition=0
  Guidance Mode Selector : Stateflow chart  TreatAsAtomicUnit=on  SystemSampleTime=0.02
      settings: PortSchema="{\"entries\":[{\"content\":{\"sides\":[{\"content\":{\"connectorIds\":[\"In1\",\"In2\",\"In3\",\"In4\",\"In5\",\"In6\",\"In7\"]},\"type\":\"ConnectorPlacement.EquallySpacedRectSide\",\"uuid\":\"a9cfd0e2-196c-422d-b359-9161a47768c9\"},{\"content\":{\"connectorIds\":[\"Out7\",\"Out2\",\"Out3\",\"Out4\",\"Out5\",\"Out6\",\"Out1\"],\"side\":\"RIGHT\"},\"type\":\"ConnectorPlacement.EquallySpacedRectSide\",\"uuid\":\"4fed41ae-e7cf-4de3-8bdb-9e24e7d8b079\"},{\"content\":{\"side\":\"TOP\"},\"type\":\"ConnectorPlacement.EquallySpacedRectSide\",\"uuid\":\"2d49ff20-2f63-498d-ac9d-820eae01f794\"}]},\"type\":\"ConnectorPlacement.EquallySpacedConnector\",\"uuid\":\"88d403f4-ad96-40f9-9697-84906f26a8bf\"}],\"packageUris\":[\"http://schema.mathworks.com/mf0/Connector/R2020b\"],\"version\":\"1.0\"}"
  Home : Constant  Value=[0 0 0]  OutDataTypeStr=double
  Landed? : simulink/Logic and Bit Operations/Compare To Constant  relop===  const=2  OutDataTypeStr=boolean
  MissionAction : Constant  Value=0  OutDataTypeStr=uint8
  Mux : Mux  Inputs=2
  Rate Transition : RateTransition
  "Select \"From\" Waypoint" : Selector  InputPortWidth=2  IndexOptions=Index vector (dialog)  Indices=2  OutputSizes=1
  "Select \"To\" Waypoint" : Selector  InputPortWidth=2  IndexOptions=Index vector (dialog)  Indices=1  OutputSizes=1
  Stop Simulation : Stop
  Takeoff IC : InitialCondition
  Terminator : Terminator
  UAV Path Manager : uavalgslib/Path Manager  UAVType=multirotor  LoiterRadius=25  dataType=double  inputBusName='doubleUavPathManager'  SimulateUsing=Code generation
  HoverCommands : Outport
  AACSP : Outport  Port=2
  FixedWingSP : Outport  Port=3
  ctrlMode : Outport  Port=4
  FlightMode : Outport  Port=5
  wires:
  Takeoff IC/1 -> Guidance Mode Selector/1(mode)
  MissionAction/1 -> UAV Path Manager/4
  Guidance Mode Selector/1(Status) -> Delay/1, Landed?/1
  Home/1 -> UAV Path Manager/5
  GCSCommands/1 -> UAV Path Manager/2
  UAV Path Manager/1 -> Rate Transition/1
  Bus Selector/1 -> Takeoff IC/1  "<mode>"
  [pose] -> Guidance Mode Selector/4(Pose)
  Compare To Constant/1 -> UAV Path Manager/3
  "Select \"To\" Waypoint"/1 -> Guidance Mode Selector/2(ToWP), Bus Selector/1
  "Select \"From\" Waypoint"/1 -> Guidance Mode Selector/3(FromWP)
  Landed?/1 -> Stop Simulation/1
  Guidance Mode Selector/2(GdncMode) -> Terminator/1
  Delay/1 -> Compare To Constant/1
  LandingStates/1 -> [landingState]
  States/1 -> Guidance Mode Selector/5(States)
  Guidance Mode Selector/5(controlMode) -> ctrlMode/1
  Guidance Mode Selector/3(aacSP) -> AACSP/1
  Guidance Mode Selector/4(FixedWingSP) -> FixedWingSP/1
  Guidance Mode Selector/6(FlightMode) -> FlightMode/1
  Constant/1 -> Guidance Mode Selector/6(PresetMode)
  "Bus "/1 -> Mux/1  "<LAP>"
  "Bus "/2 -> Mux/2  "<YawCmd>"
  Mux/1 -> HoverCommands/1
  Guidance Mode Selector/7(InnerLoopCmds) -> "Bus "/1
  Ground/1 -> Guidance Mode Selector/7(Ground)
  Pose/1 -> UAV Path Manager/1, [pose]
  Rate Transition/1 -> "Select \"From\" Waypoint"/1, "Select \"To\" Waypoint"/1

== system Alternative_VTOLAutopilotController/Guidance Test Bench/ControlType/Guidance Testbench/Guidance Logic/Interface ==
  UAVState : Inport
  Bus Creator : BusCreator  Inputs=5
  Bus Selector : BusSelector  OutputSignals=Xe,Ve
  Demux : Demux  Outputs=3
  Selector : Selector  InputPortWidth=3  IndexOptions=Index vector (dialog)  Indices=[1]  OutputSizes=1
  Selector1 : Selector  InputPortWidth=3  IndexOptions=Index vector (dialog)  Indices=[2]  OutputSizes=1
  States : Outport
  wires:
  Demux/2 -> Bus Creator/2  "y"
  UAVState/1 -> Bus Selector/1
  Bus Selector/2 -> Selector/1, Selector1/1  "<Ve>"
  Bus Selector/1 -> Demux/1  "<Xe>"
  Demux/1 -> Bus Creator/1  "x"
  Selector/1 -> Bus Creator/4  "vx"
  Demux/3 -> Bus Creator/3  "z"
  Selector1/1 -> Bus Creator/5  "vy"
  Bus Creator/1 -> States/1

== system Alternative_VTOLAutopilotController/Guidance Test Bench/ControlType/Guidance Testbench/Guidance Logic/Subsystem ==
  note: Tilt Angle also determines the state aircraft is in. Thus a unit delay is added
  UAVState : Inport
  Bus Creator : BusCreator  Inputs=6  OutDataTypeStr=Bus: GuidanceStates
  Bus Selector : BusSelector  OutputSignals=Euler,pqr,Ve,Xe,course,RotorParameters.Tilt1
  Gain : Gain
  Unit Delay : UnitDelay  InitialCondition=tiltIni  SampleTime=-1
  States : Outport
  wires:
  UAVState/1 -> Bus Selector/1
  Bus Selector/1 -> Bus Creator/1  "<Euler>"
  Bus Creator/1 -> States/1
  Bus Selector/3 -> Bus Creator/3  "<Ve>"
  Bus Selector/2 -> Bus Creator/2  "<pqr>"
  Bus Selector/4 -> Bus Creator/4  "<Xe>"
  Bus Selector/5 -> Bus Creator/5  "<course>"
  Gain/1 -> Bus Creator/6  "Tilt"
  Unit Delay/1 -> Gain/1  "Tilt1"
  Bus Selector/6 -> Unit Delay/1  "<Tilt1>"

== system Alternative_VTOLAutopilotController/Guidance Test Bench/ControlType/Manual Control/Command Interface/Control Rate Transition ==
  FM : Inport
  "ControlMode " : Inport  Port=2
  FixedWingSetpoint : Inport  Port=3
  AACSetpoint : Inport  Port=4
  Position : Inport  Port=5
  Rate Transition{,1..3,5} (5 alike) : RateTransition  OutPortSampleTime=ControlSampleTime
  ctrlMode : Outport
  FixedWingSP : Outport  Port=2
  AACSP : Outport  Port=3
  PositionCmds : Outport  Port=4
  FlightMode : Outport  Port=5
  wires:
  Rate Transition5/1 -> FlightMode/1
  Position/1 -> Rate Transition3/1
  FixedWingSetpoint/1 -> Rate Transition1/1
  Rate Transition3/1 -> PositionCmds/1
  FM/1 -> Rate Transition5/1
  "ControlMode "/1 -> Rate Transition/1
  Rate Transition1/1 -> FixedWingSP/1
  AACSetpoint/1 -> Rate Transition2/1
  Rate Transition2/1 -> AACSP/1
  Rate Transition/1 -> ctrlMode/1

== system Alternative_VTOLAutopilotController/Guidance Test Bench/ControlType/Manual Control/Command Interface/Subsystem ==
  note: Tilt Angle also determines the state aircraft is in. Thus a unit delay is added
  UAVState : Inport
  Bus Creator : BusCreator  Inputs=6  OutDataTypeStr=Bus: GuidanceStates
  Bus Selector : BusSelector  OutputSignals=Euler,pqr,Ve,Xe,course,RotorParameters.Tilt1
  Gain : Gain
  Unit Delay : UnitDelay  InitialCondition=tiltIni  SampleTime=-1
  States : Outport
  wires:
  UAVState/1 -> Bus Selector/1
  Bus Selector/1 -> Bus Creator/1  "<Euler>"
  Bus Creator/1 -> States/1
  Bus Selector/3 -> Bus Creator/3  "<Ve>"
  Bus Selector/2 -> Bus Creator/2  "<pqr>"
  Bus Selector/4 -> Bus Creator/4  "<Xe>"
  Bus Selector/5 -> Bus Creator/5  "<course>"
  Bus Selector/6 -> Unit Delay/1  "<Tilt1>"
  Gain/1 -> Bus Creator/6  "Tilt"
  Unit Delay/1 -> Gain/1  "Tilt2"

== system Alternative_VTOLAutopilotController/Low level controller/Fixed Wing Controller/Fixed Wing Controller Module/Fixed Wing Controller Simulation/AER from Path Manager ==
  In1 : Inport
  Enable : EnablePort
  Out1 : Outport
  wires:
  In1/1 -> Out1/1

== system Alternative_VTOLAutopilotController/Low level controller/Fixed Wing Controller/Fixed Wing Controller Module/Fixed Wing Controller Simulation/Airspeed-Altitude Controller ==
  note: Airspeed and altitude are controlled independently
      | by ignoring their coupled dynamics.
  Airspeed SP : Inport
  Altitude SP : Inport  Port=2
  Climb Rate SP : Inport  Port=3
  Airspeed : Inport  Port=4
  xyz : Inport  Port=5
  vxyz : Inport  Port=6
  Enable : EnablePort  ShowOutputPort=on
  Airspeed Controller : slpidlib/PID Controller  Controller=PID  Form=Parallel  TimeDomain=Discrete-time  UseExternalTs=off  SampleTime=ControlSampleTime  IntegratorMethod=Trapezoidal  FilterMethod=Forward Euler  ControllerParametersSource=internal  P=FWControlParams.P_AIRSPD  I=FWControlParams.I_AIRSPD  UseKiTs=off  D=FWControlParams.D_AIRSPD  UseExternalDerivativeSource=off  N=FWControlParams.N_AIRSPD  UseFilter=on  TunerSelectOption=Transfer Function Based (PID Tuner App)  InitialConditionSource=internal  InitialConditionForIntegrator=0  InitialConditionForFilter=0  DifferentiatorICPrevScaledInput=0  ExternalReset=none  TrackingMode=off  Kt=1  LimitOutput=off  SatLimitsSource=internal  UpperSaturationLimit=Inf  LowerSaturationLimit=0  LinearizeAsGain=on  AntiWindupMode=clamping  Kb=1  LimitIntegrator=off  UpperIntegratorSaturationLimit=inf  LowerIntegratorSaturationLimit=-inf  POutMin=[]  POutMax=[]  IOutMin=[]  IOutMax=[]  DOutMin=[]  DOutMax=[]  NOutMin=[]  NOutMax=[]  SumOutMin=[]  SumOutMax=[]  SaturationOutMin=[]  SaturationOutMax=[]  PParamMin=[]  PParamMax=[]  IParamMin=[]  IParamMax=[]  DParamMin=[]  DParamMax=[]  NParamMin=[]  NParamMax=[]  KbParamMin=[]  KbParamMax=[]  KtParamMin=[]  KtParamMax=[]  KbOutMin=[]  KbOutMax=[]  KtOutMin=[]  KtOutMax=[]  IntegratorOutMin=[]  IntegratorOutMax=[]  FilterOutMin=[]  FilterOutMax=[]  SumI1OutMin=[]  SumI1OutMax=[]  SumI2OutMin=[]  SumI2OutMax=[]  SumI3OutMin=[]  SumI3OutMax=[]  SumI4OutMin=[]  SumI4OutMax=[]  SumDOutMin=[]  SumDOutMax=[]  DifferentiatorOutMin=[]  DifferentiatorOutMax=[]  FilterDiffOutCoefMin=[]  FilterDiffOutCoefMax=[]  ReciprocalOutMin=[]  ReciprocalOutMax=[]  SumDenOutMin=[]  SumDenOutMax=[]  SumNumOutMin=[]  SumNumOutMax=[]  DivideOutMin=[]  DivideOutMax=[]  UdiffTsProdOutMin=[]  UdiffTsProdOutMax=[]  NTsProdOutMin=[]  NTsProdOutMax=[]  UintegralTsProdOutMin=[]  UintegralTsProdOutMax=[]  UngainTsProdOutMin=[]  UngainTsProdOutMax=[]  ClampingZeroOutDataTypeStr=Inherit: Inherit via back propagation  ClampingZeroOutMin=[]  ClampingZeroOutMax=[]  FilterDenConstantOutDataTypeStr=Inherit: Inherit via back propagation  FilterDenConstantOutMin=[]  FilterDenConstantOutMax=[]  PCopyOutDataTypeStr=Inherit: Inherit via back propagation  PCopyOutMin=[]  PCopyOutMax=[]  NCopyOutDataTypeStr=Inherit: Inherit via back propagation  NCopyOutMin=[]  NCopyOutMax=[]  IntegratorContinuousStateAttributes=''  IntegratorStateMustResolveToSignalObject=off  IntegratorRTWStateStorageClass=Auto  FilterContinuousStateAttributes=''  FilterStateMustResolveToSignalObject=off  FilterRTWStateStorageClass=Auto  ParallelPVariant=InternalParameters  IdealPVariant=Disabled  IVariant=InternalParameters  DVariant=InternalParameters  IntegratorVariant=Discrete  SatVariant=Disabled  AWVariant=Passthrough  PCopyVariant=Disabled  TRVariant=Disabled  FdbkBlocksVariant=Forward  IdealPFdbkVariant=Disabled  SatFdbkVariant=Disabled  DerivativeFilterVariant=ForwardEulerFilter  NVariant=InternalParameters  NCopyVariant=Disabled  FilterICVariant=InternalICsFilter  IntegratorICVariant=InternalICs  ExternalResetVariant=Disabled  TRSumVariant=Passthrough  SumFdbkVariant=Disabled  SumVariant=Sum_PID  TsampFilterVariant=InternalTs  TsampNgainVariant=Passthrough  TsampIntegralVariant=Disabled_SignalSpec  ExternalSaturationOutDataTypeStr=Inherit: Same as second input  DerivativeSourceVariant=ErrorSignal  PreIntVariant=InternalPreInt
  Altitude controller : Subsystem
  Climb Rate SP Merge : Merge
  Climb Rate SP from Guidance : Subsystem  TreatAsAtomicUnit=on
  Compare To Constant : simulink/Logic and Bit Operations/Compare To Constant  relop===  const=uint8(1)  OutDataTypeStr=boolean
  Compare To Constant1 : simulink/Logic and Bit Operations/Compare To Constant  relop===  const=uint8(2)  OutDataTypeStr=boolean
  Pitch SP Controller : Subsystem
  Sum1 : Sum  Inputs=|+-
  Pitch SP : Outport
  Throttle : Outport  Port=2
  wires:
  Airspeed SP/1 -> Sum1/1
  Sum1/1 -> Airspeed Controller/1
  Airspeed/1 -> Sum1/2
  Airspeed Controller/1 -> Throttle/1
  Altitude SP/1 -> Altitude controller/1(Alt SP)
  xyz/1 -> Altitude controller/2(xyz)
  vxyz/1 -> Pitch SP Controller/2(vxyz)
  Pitch SP Controller/1(Pitch SP) -> Pitch SP/1
  Enable/1 -> Compare To Constant1/1, Compare To Constant/1
  Compare To Constant/1 -> Altitude controller/Enable
  Compare To Constant1/1 -> Climb Rate SP from Guidance/Enable
  Altitude controller/1(Climb Rate SP) -> Climb Rate SP Merge/1
  Climb Rate SP from Guidance/1(Out1) -> Climb Rate SP Merge/2
  Climb Rate SP Merge/1 -> Pitch SP Controller/1(Climb Rate SP)
  Climb Rate SP/1 -> Climb Rate SP from Guidance/1(Climb Rate SP)

== system Alternative_VTOLAutopilotController/Low level controller/Fixed Wing Controller/Fixed Wing Controller Module/Fixed Wing Controller Simulation/Attitude Controller ==
  YPR SP : Inport
  ypr : Inport  Port=2
  Ang Rate : Inport  Port=3
  Airspeed : Inport  Port=4
  Enable : EnablePort  ShowOutputPort=on
  AER Merge : Merge
  Compare To Constant : simulink/Logic and Bit Operations/Compare To Constant  relop===  const=uint8(1)  OutDataTypeStr=boolean
  Compare To Constant1 : simulink/Logic and Bit Operations/Compare To Constant  relop===  const=uint8(2)  OutDataTypeStr=boolean
  Demux1 : Demux  Outputs=3
  Pitch Roll Controller : Subsystem
  Rudder Heading Controller : Subsystem
  AER : Outport
  wires:
  ypr/1 -> Rudder Heading Controller/2(YPR), Pitch Roll Controller/3(YPR)
  YPR SP/1 -> Demux1/1
  Enable/1 -> Compare To Constant1/1, Compare To Constant/1
  AER Merge/1 -> AER/1
  Compare To Constant/1 -> Pitch Roll Controller/Enable
  Pitch Roll Controller/1(AER) -> AER Merge/1
  Rudder Heading Controller/1(AER) -> AER Merge/2
  Demux1/1 -> Rudder Heading Controller/1(Yaw SP)
  Demux1/2 -> Pitch Roll Controller/1(Pitch SP)
  Demux1/3 -> Pitch Roll Controller/2(Roll SP)
  Ang Rate/1 -> Rudder Heading Controller/3(Ang Rate), Pitch Roll Controller/4(Ang Rate)
  Compare To Constant1/1 -> Rudder Heading Controller/Enable
  Airspeed/1 -> Pitch Roll Controller/5(Airspeed)

== system Alternative_VTOLAutopilotController/Low level controller/Fixed Wing Controller/Fixed Wing Controller Module/Fixed Wing Controller Simulation/Lateral Guidance Logic ==
  note: S. Park, J. Deyst, and J. P. How, "A New Nonlinear Guidance Logic for Trajectory Tracking," Proceedings of the AIAA Guidance, Navigation and Control Conference, Aug 2004. AIAA-2004-4900.
  Course SP : Inport
  L1 Distance : Inport  Port=2
  course : Inport  Port=3
  gndspeed : Inport  Port=4
  Enable : EnablePort
  MATLAB Function : MATLAB Function  TreatAsAtomicUnit=on  SystemSampleTime=ControlSampleTime
  Terminator : Terminator
  Roll SP : Outport
  wires:
  Course SP/1 -> MATLAB Function/1(courseSP)
  course/1 -> MATLAB Function/2(course)
  MATLAB Function/2(rollSP) -> Roll SP/1
  MATLAB Function/1(lacc) -> Terminator/1
  gndspeed/1 -> MATLAB Function/3(groundSpeed)
  L1 Distance/1 -> MATLAB Function/4(L1)
